simulink library "PressureNode"  (R2018b)
settings: Solver=VariableStepAuto  StartTime=0.0  StopTime=10.0  RelTol=1e-3
undefined symbols (not defined in the file): DPConstant, DPLinear, DPQuadratic, MassFlow
libraries: carnot x5
settings Model: Creator=drhf  LastModifiedBy=P41573

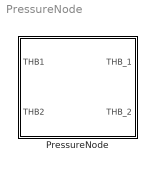
== system PressureNode ==
  PressureNode : Subsystem

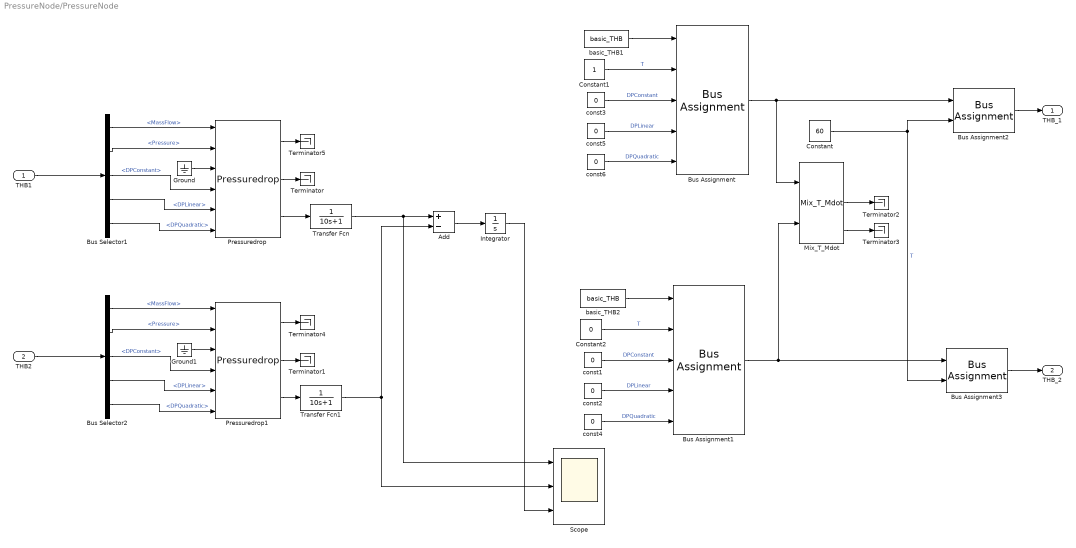
== system PressureNode/PressureNode ==
  THB1 : Inport
  THB2 : Inport  Port=2
  Add : Sum  Inputs=+-
  Bus Assignment : BusAssignment  AssignedSignals=MassFlow,DPConstant,DPLinear,DPQuadratic
  Bus Assignment1 : BusAssignment  AssignedSignals=MassFlow,DPConstant,DPLinear,DPQuadratic
  Bus Assignment2 : BusAssignment  AssignedSignals=Temperature
  Bus Assignment3 : BusAssignment  AssignedSignals=Temperature
  Bus Selector1 : BusSelector  OutputSignals=MassFlow,Pressure,DPConstant,DPLinear,DPQuadratic
  Bus Selector2 : BusSelector  OutputSignals=MassFlow,Pressure,DPConstant,DPLinear,DPQuadratic
  Constant : Constant  Value=60
  Constant1 : Constant
  Constant2 : Constant  Value=0
  Ground : Ground
  Ground1 : Ground
  Integrator : Integrator  LimitOutput=on  LowerSaturationLimit=0
  Mix_T_Mdot : carnot/Basic/Hydraulics/Mix_T_Mdot  mixcalc=Tmix = (mdot1*T1 + mdot2*T2)/(mdot1+mdot2)
      settings: SourceProductName=Carnot
  Pressuredrop : carnot/Basic/Pressure_Drop/Pressuredrop
      settings: SourceProductName=Carnot
  Pressuredrop1 : carnot/Basic/Pressure_Drop/Pressuredrop
      settings: SourceProductName=Carnot
  Scope : Scope  NumInputPorts=3
  Terminator{,1..5} (6 alike) : Terminator
  Transfer Fcn : TransferFcn  Denominator=[10 1]
  Transfer Fcn1 : TransferFcn  Denominator=[10 1]
  basic_THB1 : carnot/Basic/Hydraulics/basic_THB  t=20  mdot=0  p=1e5  ID=Pressure Drop from Massflow  fluid=Water  mix=0  mix2=0  mix3=0  dia=0.02  hgt=0
      settings: SourceProductName=Carnot
  basic_THB2 : carnot/Basic/Hydraulics/basic_THB  t=20  mdot=0  p=1e5  ID=Pressure Drop from Massflow  fluid=Water  mix=0  mix2=0  mix3=0  dia=0.02  hgt=0
      settings: SourceProductName=Carnot
  const{1..6} (6 alike) : Constant  Value=0
  THB_1 : Outport
  THB_2 : Outport  Port=2
  wires:
  const5/1 -> Bus Assignment/4  "DPLinear"
  const6/1 -> Bus Assignment/5  "DPQuadratic"
  THB1/1 -> Bus Selector1/1
  Bus Selector1/1 -> Pressuredrop/1  "<MassFlow>"
  Bus Selector1/2 -> Pressuredrop/2  "<Pressure>"
  Bus Selector1/3 -> Pressuredrop/4  "<DPConstant>"
  Bus Selector1/4 -> Pressuredrop/5  "<DPLinear>"
  Bus Selector1/5 -> Pressuredrop/6  "<DPQuadratic>"
  Ground/1 -> Pressuredrop/3
  Pressuredrop/2 -> Terminator/1
  Pressuredrop1/2 -> Terminator1/1
  Ground1/1 -> Pressuredrop1/3
  Bus Selector2/5 -> Pressuredrop1/6  "<DPQuadratic>"
  Bus Selector2/4 -> Pressuredrop1/5  "<DPLinear>"
  Bus Selector2/3 -> Pressuredrop1/4  "<DPConstant>"
  Bus Selector2/2 -> Pressuredrop1/2  "<Pressure>"
  Bus Selector2/1 -> Pressuredrop1/1  "<MassFlow>"
  THB2/1 -> Bus Selector2/1
  basic_THB1/1 -> Bus Assignment/1
  Bus Assignment1/1 -> Bus Assignment3/1, Mix_T_Mdot/2
  Add/1 -> Integrator/1
  Bus Assignment/1 -> Bus Assignment2/1, Mix_T_Mdot/1
  Bus Assignment2/1 -> THB_1/1
  Mix_T_Mdot/2 -> Terminator2/1
  Mix_T_Mdot/3 -> Terminator3/1
  Constant/1 -> Bus Assignment3/2, Bus Assignment2/2  "T"
  Bus Assignment3/1 -> THB_2/1
  const3/1 -> Bus Assignment/3  "DPConstant"
  Constant1/1 -> Bus Assignment/2  "T"
  Transfer Fcn/1 -> Scope/1, Add/1
  Transfer Fcn1/1 -> Scope/2, Add/2
  Integrator/1 -> Scope/3
  Constant2/1 -> Bus Assignment1/2  "T"
  const1/1 -> Bus Assignment1/3  "DPConstant"
  basic_THB2/1 -> Bus Assignment1/1
  const4/1 -> Bus Assignment1/5  "DPQuadratic"
  const2/1 -> Bus Assignment1/4  "DPLinear"
  Pressuredrop/1 -> Terminator5/1
  Pressuredrop/3 -> Transfer Fcn/1
  Pressuredrop1/1 -> Terminator4/1
  Pressuredrop1/3 -> Transfer Fcn1/1
